simulink model "VGrowth2"  (R2018b)
settings: Solver=VariableStepAuto  StartTime=1e-3  StopTime=12  RelTol=1e-3
libraries: simulink x2, aerolibanimutils x1
Description:
  | https://docs.iota.org/introduction/iota-token/the-iota-token
settings Model: Creator=Magneto  LastModifiedBy=Magneto
settings SolverCC: ZeroCrossAlgorithm=Adaptive
settings DebuggingCC: IgnoredZcDiagnostic=none

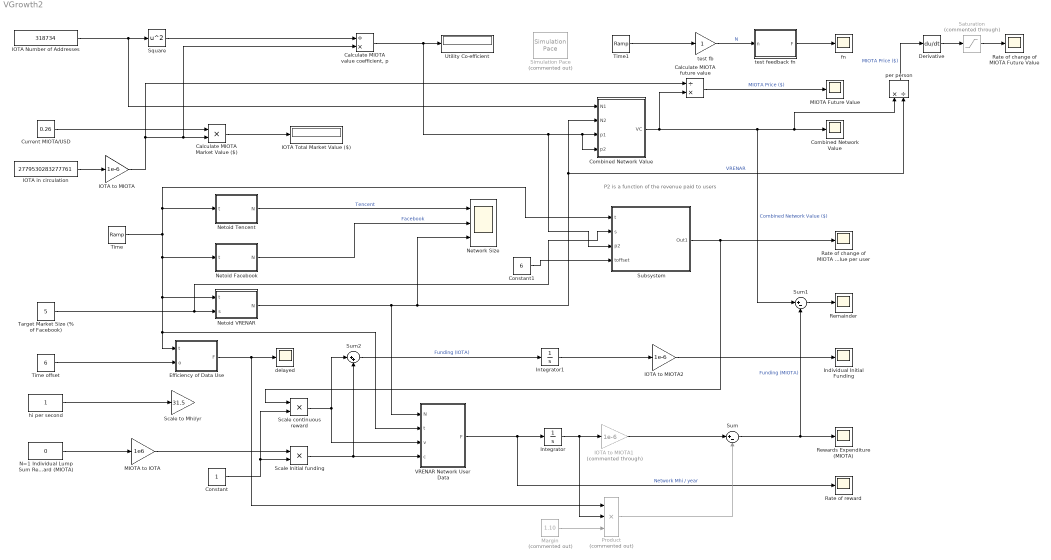
== system VGrowth2 ==
  note: P2 is a function of the revenue paid to users
  " Combined Network Value" : MATLAB Function  TreatAsAtomicUnit=on
  " per person" : Product  Inputs=*/
  Calculate MIOTA Market Value ($) : Product  Inputs=**
  Calculate MIOTA future value : Product  Inputs=/*
  "Calculate MIOTA value coefficient, p" : Product  Inputs=/*
  Combined Network Value : Scope
  Constant : Constant
  Constant1 : Constant  Value=6
  Current MIOTA/USD : Constant  Description=Value obtained from https://coinmarketcap.com/currencies/iota/  Value=0.26
  Derivative : Derivative
  Efficiency of Data Use : MATLAB Function  TreatAsAtomicUnit=on
  IOTA Number of Addresses : Constant  Value=318734
  IOTA Total Market Value ($) : Display
  IOTA in circulation : Constant  Value=2779530283277761
  IOTA to MIOTA : Gain  Gain=1e-6
  IOTA to MIOTA1 : Gain  Commented=through  Gain=1e-6
  IOTA to MIOTA2 : Gain  Gain=1e-6
  Individual Initial Funding : Scope
  Integrator : Integrator
  Integrator1 : Integrator
  MIOTA Future Value : Scope
  MIOTA to IOTA : Gain  Gain=1e6
  Margin : Constant  Commented=on  Value=1.10
  N=1 Individual Lump Sum Reward (MIOTA) : Constant  Value=0
  Netoid Facebook : MATLAB Function  TreatAsAtomicUnit=on
  Netoid Tencent : MATLAB Function  TreatAsAtomicUnit=on
  Netoid VRENAR : MATLAB Function  TreatAsAtomicUnit=on
  Network Size : Scope  NumInputPorts=3
  Product : Product  Commented=on  Inputs=3
  Rate of change of MIOTA Future Value : Scope
  Rate of change of MIOTA future Value per user : Scope
  Rate of reward : Scope
  Remainder : Scope
  Rewards Expenditure (MIOTA) : Scope
  Saturation : Saturate  Commented=through  UpperLimit=inf  LowerLimit=0
  Scale Initial funding : Product  Inputs=**
  Scale continuous reward : Product  Inputs=**
  Scale to Mhi/yr : Gain  Gain=31.5
  Simulation Pace : aerolibanimutils/Simulation Pace  Commented=on  SimulationPace=0.33333  SleepMode=Auto  OutputPaceError=off  SampleTime=1/30
  Square : Math  Operator=square  SaturateOnIntegerOverflow=on
  Subsystem : Subsystem
  Sum : Sum  Inputs=|+-
  Sum1 : Sum  Inputs=|+-
  Sum2 : Sum  Inputs=|++
  Target Market Size (% of Facebook) : Constant  Value=5
  Time : simulink/Sources/Ramp  slope=1  start=0  InitialOutput=0
  Time offset : Constant  Value=6
  Time1 : simulink/Sources/Ramp  slope=1  start=0  InitialOutput=0
  Utility Co-efficient : Display
  VRENAR Network User Data : MATLAB Function  TreatAsAtomicUnit=on
  delayed : Scope
  fn : Scope
  hi per second : Constant
  test fb : Gain
  test feedback fn : MATLAB Function  TreatAsAtomicUnit=on
  wires:
  Netoid Facebook/1(N) -> Network Size/2  "Facebook"
  Netoid Tencent/1(N) -> Network Size/1  "Tencent"
  VRENAR Network User Data/1(F) -> Rate of reward/1, Integrator/1  "Network Mhi / year"
  Netoid VRENAR/1(N) -> VRENAR Network User Data/1(N), " per person"/2, " Combined Network Value"/2(N2), Network Size/3  "VRENAR"
  Sum/1 -> Sum1/2, Rewards Expenditure (MIOTA)/1  "Funding (MIOTA)"
  Square/1 -> "Calculate MIOTA value coefficient, p"/1
  "Calculate MIOTA value coefficient, p"/1 -> Subsystem/3(p2), " Combined Network Value"/3(p1), " Combined Network Value"/4(p2), Utility Co-efficient/1
  hi per second/1 -> Scale to Mhi/yr/1
  Scale continuous reward/1 -> VRENAR Network User Data/3(v), Sum2/1
  " Combined Network Value"/1(VC) -> Calculate MIOTA future value/2, Sum1/1, " per person"/1, Combined Network Value/1  "Combined Network Value ($)"
  IOTA Number of Addresses/1 -> " Combined Network Value"/1(N1), Square/1
  IOTA in circulation/1 -> IOTA to MIOTA/1
  Current MIOTA/USD/1 -> Calculate MIOTA Market Value ($)/1
  Calculate MIOTA Market Value ($)/1 -> IOTA Total Market Value ($)/1
  Integrator/1 -> Product/2, IOTA to MIOTA1/1
  N=1 Individual Lump Sum Reward (MIOTA)/1 -> MIOTA to IOTA/1
  Scale Initial funding/1 -> Sum2/2, VRENAR Network User Data/4(c)
  MIOTA to IOTA/1 -> Scale Initial funding/1
  Calculate MIOTA future value/1 -> MIOTA Future Value/1  "MIOTA Price ($)"
  IOTA to MIOTA1/1 -> Sum/1
  Target Market Size (% of Facebook)/1 -> Subsystem/2(s), Netoid VRENAR/2(s)
  Sum2/1 -> Integrator1/1  "Funding (IOTA)"
  Integrator1/1 -> IOTA to MIOTA2/1
  IOTA to MIOTA2/1 -> Individual Initial Funding/1
  Time1/1 -> test fb/1
  test fb/1 -> test feedback fn/1(n)  "N"
  test feedback fn/1(F) -> fn/1
  IOTA to MIOTA/1 -> Calculate MIOTA future value/1, "Calculate MIOTA value coefficient, p"/2, Calculate MIOTA Market Value ($)/2
  Constant/1 -> Scale continuous reward/2, Scale Initial funding/2
  Time/1 -> Netoid Tencent/1(t), Subsystem/1(t), Netoid Facebook/1(t), Netoid VRENAR/1(t), Efficiency of Data Use/1(t), VRENAR Network User Data/2(t)
  Efficiency of Data Use/1(F) -> Product/1, delayed/1
  Margin/1 -> Product/3
  Product/1 -> Sum/2
  Time offset/1 -> Efficiency of Data Use/2(o)
  Derivative/1 -> Saturation/1
  Saturation/1 -> Rate of change of MIOTA Future Value/1
  " per person"/1 -> Derivative/1  "MIOTA Price ($)"
  Constant1/1 -> Subsystem/4(toffset)
  Subsystem/1(Out1) -> Scale continuous reward/1, Rate of change of MIOTA future Value per user/1
  Sum1/1 -> Remainder/1

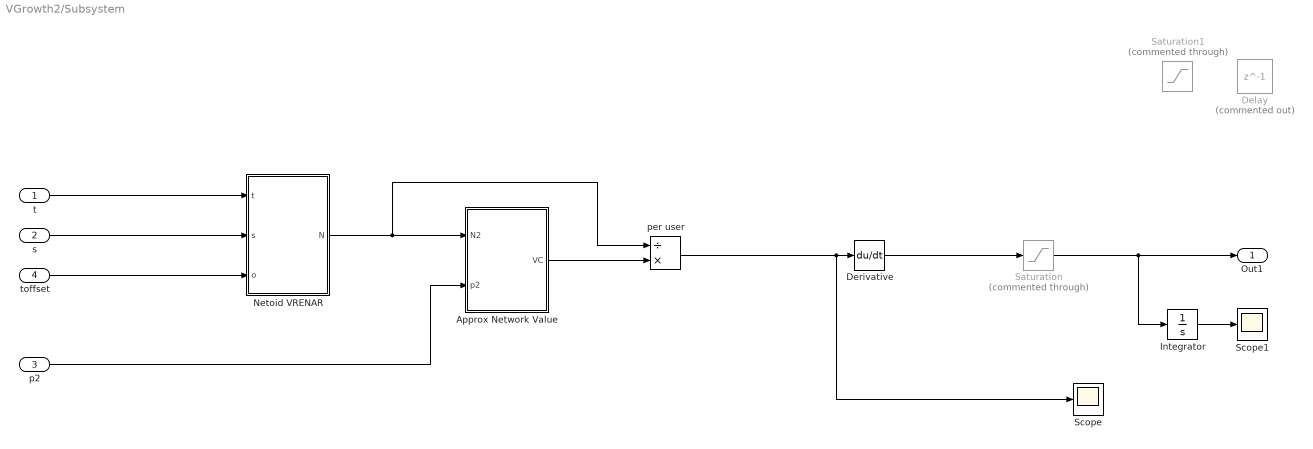
== system VGrowth2/Subsystem ==
  t : Inport
  s : Inport  Port=2
  p2 : Inport  Port=3
  toffset : Inport  Port=4
  " Approx Network Value" : MATLAB Function  TreatAsAtomicUnit=on
  " per user" : Product  Inputs=/*
  Delay : Delay  Commented=on  DelayLength=1  InitialCondition=1
  Derivative : Derivative
  Integrator : Integrator
  Netoid VRENAR : MATLAB Function  TreatAsAtomicUnit=on
  Saturation : Saturate  Commented=through  UpperLimit=inf  LowerLimit=0
  Saturation1 : Saturate  Commented=through  UpperLimit=inf  LowerLimit=1e-9
  Scope : Scope
  Scope1 : Scope
  Out1 : Outport
  wires:
  s/1 -> Netoid VRENAR/2(s)
  p2/1 -> " Approx Network Value"/2(p2)
  t/1 -> Netoid VRENAR/1(t)
  toffset/1 -> Netoid VRENAR/3(o)
  " per user"/1 -> Scope/1, Derivative/1
  Derivative/1 -> Saturation/1
  Saturation/1 -> Integrator/1, Out1/1
  " Approx Network Value"/1(VC) -> " per user"/2
  Netoid VRENAR/1(N) -> " per user"/1, " Approx Network Value"/1(N2)
  Integrator/1 -> Scope1/1

== matlab function VGrowth2/Netoid Tencent ==
  data: t input; N output
function N = fcn(t)

N = 2.61e9/(1+exp(-0.3*(t-10)));

== matlab function VGrowth2/VRENAR Network User Data ==
  data: N input; t input; F output; v input; c input
function F = fcn(N,t,v,c)

F = N*(c+(v*t));

== matlab function VGrowth2/Netoid Facebook ==
  data: t input; N output
function N = fcn(t)

N = 1.45e9/(1+exp(-0.77*(t-5)));

== matlab function VGrowth2/Netoid VRENAR ==
  data: t input; N output; s input
function N = fcn(t,s)

% Additional term -(1.45e9/(1+exp(-1.155*(-5)))) added to initialise N
% closer to zero at t=0
N = (s/100)*((1.45e9/(1+exp(-1.155*(t-5))))-(1.45e9/(1+exp(-1.155*(-5)))));

== matlab function VGrowth2/Subsystem/Netoid VRENAR ==
  data: t input; N output; s input; o input
function N = fcn(t,s,o)

% Additional term -(1.45e9/(1+exp(-1.155*(-5)))) added to initialise N
% closer to zero at t=0
N = (s/100)*((1.45e9/(1+exp(-1.155*(t-o))))-(1.45e9/(1+exp(-1.155*(-o)))));

== matlab function VGrowth2/ Combined Network Value ==
  data: N1 input; N2 input; VC output; p1 input; p2 input
function VC = fcn(N1,N2,p1,p2)

VC = (p1*N1^2+2*N1*N2*(p1+p2)+p2*N2^2);

== matlab function VGrowth2/test feedback fn ==
  data: n input; F output
function F = fcn(n)

% F = n/2e7*(1-1/(1+exp(n)));
% F = 1e-12*n^3;
F = 1/(1*(1+exp((n-5)*1.55)));

== matlab function VGrowth2/Efficiency of Data Use ==
  data: t input; F output; o input
function F = fcn(t,o)

% Additional term -(1.45e9/(1+exp(-1.155*(-5)))) added to initialise N
% closer to zero at t=0
%F = ((1/(1+exp(-1.155*(t-o))))-(1/(1+exp(-1.155*(-o)))));
F = 1-((1/(1+exp(-1.155*(t-o))))-(1/(1+exp(-1.155*(-o)))));
%if (t <= 0.5)
%    F = 0.2;
%elseif (t > 0.5)&&(t <= 1)
%    F = 0.6;
%elseif (t > 1)
%    F = 0.95;
%else
%    F = 1;
%end

== matlab function VGrowth2/Subsystem/ Approx Network Value ==
  data: N2 input; VC output; p2 input
function VC = fcn(N2,p2)

VC = p2*N2^2;
